simulink model "BuckyWagon_01"  (Simulink 7.5)
settings: Solver=FixedStepDiscrete  StartTime=0.0  StopTime=10.0  RelTol=1e-3
PreLoadFcn:
  | try, eval([bdroot '_setup']); catch, eval('model_setup', ''); end
InitFcn:
  | try, eval([bdroot '_setup']); catch, eval('model_setup', ''); end
undefined symbols (not defined in the file): ECU565, High, Low, miniviewSetup, motohawk_build_version, motohawk_get_faults, motohawk_setup_toolchains, motohawk_trunc_name, motohawk_vardec_config_group, motohawk_vardec_path, tc, True
libraries: MotoHawk_lib x381, simulink x26, miniview_lib x10, motohawk_control_primitives_lib x8, motohawk_engine_lib x6, motohawk_annotations_lib x2
(part 2 of 6)

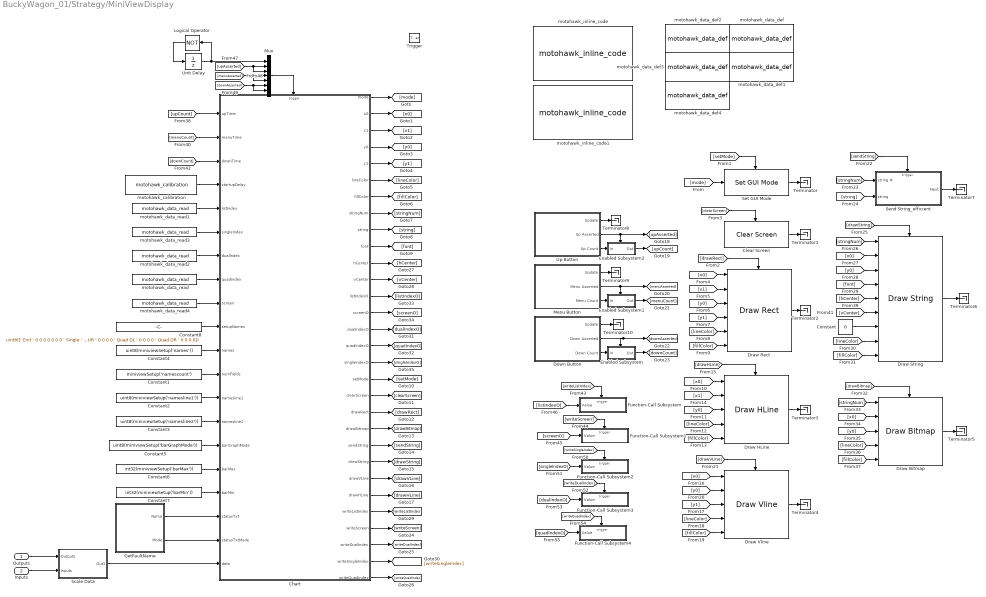
== system BuckyWagon_01/Strategy/MiniViewDisplay ==
  Outputs : Inport  OutDataType=sfix(16)  OutScaling=2^0
  Inputs : Inport  Port=2  OutDataType=sfix(16)  OutScaling=2^0
  Trigger : TriggerPort  TriggerType=function-call
  Chart : Stateflow chart  TreatAsAtomicUnit=on
      settings: RTWSystemCode=Reusable function
  Clear Screen : miniview_lib/Clear Screen  SystemSampleTime=-1  miniview_CAN_channel=1
  Constant : Constant  Value=0  OutDataType=sfix(16)  OutScaling=2^0  OutDataTypeStr=Inherit: Inherit via back propagation
  Constant1 : Constant  Value=miniviewSetup('namescount')  OutDataTypeMode=uint8  OutDataType=sfix(16)  OutScaling=2^0  OutDataTypeStr=uint8
  Constant2 : Constant  Value=uint8(miniviewSetup('namesline1'))  OutDataTypeMode=uint8  OutDataType=sfix(16)  OutScaling=2^0  OutDataTypeStr=uint8
  Constant3 : Constant  Value=uint8(miniviewSetup('namesline2'))  OutDataTypeMode=uint8  OutDataType=sfix(16)  OutScaling=2^0  OutDataTypeStr=uint8
  Constant4 : Constant  Value=uint8(miniviewSetup('names'))  OutDataTypeMode=uint8  OutDataType=sfix(16)  OutScaling=2^0  OutDataTypeStr=uint8
  Constant5 : Constant  Value=uint8(miniviewSetup('barGraphMode'))  OutDataTypeMode=uint8  OutDataType=sfix(16)  OutScaling=2^0  OutDataTypeStr=uint8
  Constant6 : Constant  Value=int32(miniviewSetup('barMax'))  OutDataTypeMode=int32  OutDataType=sfix(16)  OutScaling=2^0  OutDataTypeStr=int32
  Constant7 : Constant  Value=int32(miniviewSetup('barMin'))  OutDataTypeMode=int16  OutDataType=sfix(16)  OutScaling=2^0  OutDataTypeStr=int16
  Constant8 : Constant  Value=uint8([' Exit ' 0 0 0 0 0 0 0 ' Single ' 0 0 0 0 0 ' Dual Upper ' 0 ' Dual Lower ' 0 ' Quad UL ' 0 0 0 0 ' Quad UR ' 0 0 0 0 ' Quad DL ' 0 0 0 0 ' Quad DR ' 0 0 0 0])  OutDataTypeMode=uint8  OutDataType=sfix(16)  OutScaling=2^0  OutDataTypeStr=uint8
  Down Button : Subsystem  AncestorBlock=miniview_lib/Down Button  mask(MotoHawk MiniView Down Button){miniview_CAN_channel=1}
      mask prompts: miniview_CAN_channel "Physical CAN Channel"
      mask help: MotoHawk MiniView Down Button
      mask Display: disp(['MiniView "Down" Button\n\nChannel:  CAN_' num2str(miniview_CAN_channel)])
  Draw Bitmap : miniview_lib/Draw Bitmap  SystemSampleTime=-1  miniview_CAN_channel=1
  Draw HLine : miniview_lib/Draw HLine  SystemSampleTime=-1  miniview_CAN_channel=1
  Draw Rect : miniview_lib/Draw Rect  SystemSampleTime=-1  miniview_CAN_channel=1
  Draw String : miniview_lib/Draw String  SystemSampleTime=-1  miniview_CAN_channel=1
  Draw Vline : miniview_lib/Draw Vline  SystemSampleTime=-1  miniview_CAN_channel=1
  Enabled Subsystem : Subsystem  TreatAsAtomicUnit=on
  Enabled Subsystem1 : Subsystem  TreatAsAtomicUnit=on
  Enabled Subsystem2 : Subsystem  TreatAsAtomicUnit=on
  Function-Call Subsystem : Subsystem  TreatAsAtomicUnit=on
  Function-Call Subsystem1 : Subsystem  TreatAsAtomicUnit=on
  Function-Call Subsystem2 : Subsystem  TreatAsAtomicUnit=on
  Function-Call Subsystem3 : Subsystem  TreatAsAtomicUnit=on
  Function-Call Subsystem4 : Subsystem  TreatAsAtomicUnit=on
  GetFaultName : Subsystem
  Logical Operator : Logic  Operator=NOT  AllPortsSameDT=off  OutDataTypeMode=boolean  OutDataTypeStr=boolean
  Menu Button : Subsystem  AncestorBlock=miniview_lib/Menu Button  mask(MotoHawk MiniView Menu Button){miniview_CAN_channel=1}
      mask prompts: miniview_CAN_channel "Physical CAN Channel"
      mask help: MotoHawk MiniView Menu Button
      mask Display: disp(['MiniView "Menu" Button\n\nChannel:  CAN_' num2str(miniview_CAN_channel)])
  Mux : Mux  Inputs=7
  Scale Data : Subsystem
  Send String_efficient : Subsystem  AncestorBlock=miniview_lib/Send String  mask(MotoHawk MiniView Send String){miniview_CAN_channel=1}
      mask prompts: miniview_CAN_channel "Physical CAN Channel"
      mask help:
      | MotoHawk MiniView Send String
      |
      | Send string (#0 to #15) to gauge.
      mask Display: disp(['MiniView\nSend String\nChannel:  CAN_' num2str(miniview_CAN_channel)])
  Set GUI Mode : miniview_lib/Set GUI Mode  SystemSampleTime=-1  miniview_CAN_channel=1
  Terminator{,1..10} (11 alike) : Terminator
  Unit Delay : UnitDelay  SampleTime=-1
  Up Button : Subsystem  AncestorBlock=miniview_lib/Up Button  mask(MotoHawk MiniView Up Button){miniview_CAN_channel=1}
      mask prompts: miniview_CAN_channel "Physical CAN Channel"
      mask help: MotoHawk MiniView Up Button
      mask Display: disp(['MiniView "Up" Button\n\nChannel:  CAN_' num2str(miniview_CAN_channel)])
  motohawk_calibration : MotoHawk_lib/Calibration & Probing Blocks/motohawk_calibration  nam='startupDelay'  val=300  storage=Calibration  show_more=on  name_source=Use Parameter  data_type=uint16  read_level=1  write_level=1  ovr_cals=on  view_as=Number  enum_struct={'Disabled', 'Enabled'}  vector_style=Wide Row  use_help_units=on  help='Time to wait before drawing on the miniview.'  units='s'  use_header_enum=off  row_header_enum={}  col_header_enum={}  use_min_max=on  min_val=0  max_val=10  use_precision=on  precision='1.3'  gain=0.005  offset=0  exp=1  use_mototune_group=off  mototune_group=motohawk_vardec_path(gcb)
  motohawk_data_def : MotoHawk_lib/Data Storage Blocks/motohawk_data_def  nam='quadIndex'  container_nam=''  data=[0 5 16 19]  typ=uint8  struct_nam='MyStruct'  storage=NonVolatile  outputRef=off  use_vardec=on  window=Display  read_level=1  write_level=1  ovr_cals=on  view_as=Number  enum_struct={'Disabled', 'Enabled'}  vector_style=Tall Column  use_help_units=on  help=''  units=''  use_header_enum=off  row_header_enum=''  col_header_enum=''  use_min_max=off  min_val=-inf  max_val=inf  use_precision=off  precision=''  gain=1  offset=0  exp=1  use_mototune_group=off  mototune_group=motohawk_vardec_path(gcb)  eval_name=quadIndex  data_stores=motohawk_sfun_data_def_data_stores  struct_instances=motohawk_sfun_data_def_struct_instances  vardecs=motohawk_sfun_data_def_vardecs
  motohawk_data_def1 : MotoHawk_lib/Data Storage Blocks/motohawk_data_def  nam='listIndex'  container_nam=''  data=0  typ=uint8  struct_nam='MyStruct'  storage=NonVolatile  outputRef=off  use_vardec=on  window=Display  read_level=1  write_level=1  ovr_cals=on  view_as=Number  enum_struct={'Disabled', 'Enabled'}  vector_style=Tall Column  use_help_units=on  help=''  units=''  use_header_enum=off  row_header_enum=''  col_header_enum=''  use_min_max=off  min_val=-inf  max_val=inf  use_precision=off  precision=''  gain=1  offset=0  exp=1  use_mototune_group=off  mototune_group=motohawk_vardec_path(gcb)  eval_name=listIndex  data_stores=motohawk_sfun_data_def_data_stores  struct_instances=motohawk_sfun_data_def_struct_instances  vardecs=motohawk_sfun_data_def_vardecs
  motohawk_data_def2 : MotoHawk_lib/Data Storage Blocks/motohawk_data_def  nam='dualIndex'  container_nam=''  data=[10 27]  typ=uint8  struct_nam='MyStruct'  storage=NonVolatile  outputRef=off  use_vardec=on  window=Display  read_level=1  write_level=1  ovr_cals=on  view_as=Number  enum_struct={'Disabled', 'Enabled'}  vector_style=Tall Column  use_help_units=on  help=''  units=''  use_header_enum=off  row_header_enum=''  col_header_enum=''  use_min_max=off  min_val=-inf  max_val=inf  use_precision=off  precision=''  gain=1  offset=0  exp=1  use_mototune_group=off  mototune_group=motohawk_vardec_path(gcb)  eval_name=dualIndex  data_stores=motohawk_sfun_data_def_data_stores  struct_instances=motohawk_sfun_data_def_struct_instances  vardecs=motohawk_sfun_data_def_vardecs
  motohawk_data_def3 : MotoHawk_lib/Data Storage Blocks/motohawk_data_def  nam='singleIndex'  container_nam=''  data=15  typ=uint8  struct_nam='MyStruct'  storage=NonVolatile  outputRef=off  use_vardec=on  window=Display  read_level=1  write_level=1  ovr_cals=on  view_as=Number  enum_struct={'Disabled', 'Enabled'}  vector_style=Tall Column  use_help_units=on  help=''  units=''  use_header_enum=off  row_header_enum=''  col_header_enum=''  use_min_max=off  min_val=-inf  max_val=inf  use_precision=off  precision=''  gain=1  offset=0  exp=1  use_mototune_group=off  mototune_group=motohawk_vardec_path(gcb)  eval_name=singleIndex  data_stores=motohawk_sfun_data_def_data_stores  struct_instances=motohawk_sfun_data_def_struct_instances  vardecs=motohawk_sfun_data_def_vardecs
  motohawk_data_def4 : MotoHawk_lib/Data Storage Blocks/motohawk_data_def  nam='screen'  container_nam=''  data=0  typ=uint8  struct_nam='MyStruct'  storage=NonVolatile  outputRef=off  use_vardec=on  window=Display  read_level=1  write_level=1  ovr_cals=on  view_as=Number  enum_struct={'Disabled', 'Enabled'}  vector_style=Tall Column  use_help_units=on  help=''  units=''  use_header_enum=off  row_header_enum=''  col_header_enum=''  use_min_max=off  min_val=-inf  max_val=inf  use_precision=off  precision=''  gain=1  offset=0  exp=1  use_mototune_group=off  mototune_group=motohawk_vardec_path(gcb)  eval_name=screen  data_stores=motohawk_sfun_data_def_data_stores  struct_instances=motohawk_sfun_data_def_struct_instances  vardecs=motohawk_sfun_data_def_vardecs
  motohawk_data_read : MotoHawk_lib/Data Storage Blocks/motohawk_data_read  source=Lookup By Name  structure=Vector  operation=Read entire data structure at once  sz_vec=4  sz_row=2  sz_col=3  typ=uint8  nam='quadIndex'  checkNull=on  struct_inst_name='Struct1'  struct_nam='MyStruct'
  motohawk_data_read1 : MotoHawk_lib/Data Storage Blocks/motohawk_data_read  source=Lookup By Name  structure=Scalar  operation=Read scalar from location by index  sz_vec=4  sz_row=2  sz_col=3  typ=uint8  nam='listIndex'  checkNull=on  struct_inst_name='Struct1'  struct_nam='MyStruct'
  motohawk_data_read2 : MotoHawk_lib/Data Storage Blocks/motohawk_data_read  source=Lookup By Name  structure=Vector  operation=Read entire data structure at once  sz_vec=2  sz_row=2  sz_col=3  typ=uint8  nam='dualIndex'  checkNull=on  struct_inst_name='Struct1'  struct_nam='MyStruct'
  motohawk_data_read3 : MotoHawk_lib/Data Storage Blocks/motohawk_data_read  source=Lookup By Name  structure=Scalar  operation=Read scalar from location by index  sz_vec=4  sz_row=2  sz_col=3  typ=uint8  nam='singleIndex'  checkNull=on  struct_inst_name='Struct1'  struct_nam='MyStruct'
  motohawk_data_read4 : MotoHawk_lib/Data Storage Blocks/motohawk_data_read  source=Lookup By Name  structure=Scalar  operation=Read entire data structure at once  sz_vec=4  sz_row=2  sz_col=3  typ=uint8  nam='screen'  checkNull=on  struct_inst_name='Struct1'  struct_nam='MyStruct'
  motohawk_inline_code : MotoHawk_lib/Extra Development Blocks/motohawk_inline_code  include_code='#include <stdio.h>'  start_code=''  output_code=''
  motohawk_inline_code1 : MotoHawk_lib/Extra Development Blocks/motohawk_inline_code  include_code='#define charPtr(p) ((char*)p)'  start_code=''  output_code=''
  wires:
  Outputs/1 -> Scale Data/1(Outputs)
  Inputs/1 -> Scale Data/2(Inputs)
  Chart/1(mode) -> [mode]
  Chart/2(x0) -> [x0]
  Chart/3(x1) -> [x1]
  Chart/4(y0) -> [y0]
  Chart/5(y1) -> [y1]
  Chart/6(lineColor) -> [lineColor]
  Chart/7(fillColor) -> [fillColor]
  Chart/8(stringNum) -> [stringNum]
  Chart/9(string) -> [string]
  Chart/10(font) -> [font]
  Chart/19(clearScreen) -> [clearScreen]
  Chart/20(drawRect) -> [drawRect]
  Chart/21(drawBitmap) -> [drawBitmap]
  Chart/22(sendString) -> [sendString]
  Chart/23(drawString) -> [drawString]
  Chart/24(drawVLine) -> [drawVLine]
  Chart/25(drawHLine) -> [drawHLine]
  [setMode] -> Set GUI Mode/Trigger
  [mode] -> Set GUI Mode/1
  Set GUI Mode/1 -> Terminator/1
  [clearScreen] -> Clear Screen/Trigger
  Clear Screen/1 -> Terminator1/1
  [drawRect] -> Draw Rect/Trigger
  [x0] -> Draw Rect/1
  [x1] -> Draw Rect/2
  [y0] -> Draw Rect/3
  [y1] -> Draw Rect/4
  [lineColor] -> Draw Rect/5
  [fillColor] -> Draw Rect/6
  [x0] -> Draw HLine/1
  [x1] -> Draw HLine/2
  [y0] -> Draw HLine/3
  [lineColor] -> Draw HLine/4
  [fillColor] -> Draw HLine/5
  [drawHLine] -> Draw HLine/Trigger
  [x0] -> Draw Vline/1
  [y0] -> Draw Vline/2
  [y1] -> Draw Vline/3
  [lineColor] -> Draw Vline/4
  [fillColor] -> Draw Vline/5
  [drawVLine] -> Draw Vline/Trigger
  Draw Rect/1 -> Terminator2/1
  Draw Vline/1 -> Terminator4/1
  Draw HLine/1 -> Terminator3/1
  [sendString] -> Send String_efficient/Trigger
  [stringNum] -> Send String_efficient/1(string #)
  [string] -> Send String_efficient/2(string)
  [drawString] -> Draw String/Trigger
  [stringNum] -> Draw String/1
  [x0] -> Draw String/2
  [y0] -> Draw String/3
  [font] -> Draw String/4
  [lineColor] -> Draw String/8
  [fillColor] -> Draw String/9
  [drawBitmap] -> Draw Bitmap/Trigger
  [stringNum] -> Draw Bitmap/1
  [x0] -> Draw Bitmap/2
  [y0] -> Draw Bitmap/3
  [lineColor] -> Draw Bitmap/4
  [fillColor] -> Draw Bitmap/5
  Draw Bitmap/1 -> Terminator5/1
  Draw String/1 -> Terminator6/1
  Send String_efficient/1(Next) -> Terminator7/1
  [upCount] -> Chart/1(upTime)
  [menuCount] -> Chart/2(menuTime)
  [downCount] -> Chart/3(downTime)
  Up Button/2(Up Asserted) -> [upAsserted], Enabled Subsystem2/Enable
  Down Button/2(Down Asserted) -> [downAsserted], Enabled Subsystem/Enable
  Menu Button/2(Menu Asserted) -> [menuAsserted], Enabled Subsystem1/Enable
  [upAsserted] -> Mux/2, Mux/3
  [menuAsserted] -> Mux/4, Mux/5
  [downAsserted] -> Mux/6, Mux/7
  Mux/1 -> Chart/Trigger
  Constant/1 -> Draw String/7
  [hCenter] -> Draw String/5
  [vCenter] -> Draw String/6
  Chart/11(hCenter) -> [hCenter]
  Chart/12(vCenter) -> [vCenter]
  Unit Delay/1 -> Mux/1, Logical Operator/1
  Constant4/1 -> Chart/11(names)
  Logical Operator/1 -> Unit Delay/1
  Scale Data/1(Out1) -> Chart/20(data)
  Constant2/1 -> Chart/13(namesline1)
  Constant3/1 -> Chart/14(namesline2)
  motohawk_data_read1/1 -> Chart/5(listIndex)
  motohawk_data_read/1 -> Chart/8(quadIndex)
  Chart/26(writeListIndex) -> [writeListIndex]
  [writeListIndex] -> Function-Call Subsystem/Trigger
  motohawk_data_read2/1 -> Chart/7(dualIndex)
  motohawk_data_read3/1 -> Chart/6(singleIndex)
  Constant5/1 -> Chart/15(barGraphMode)
  Constant6/1 -> Chart/16(barMax)
  Constant7/1 -> Chart/17(barMin)
  Up Button/1(Update) -> Terminator8/1
  Menu Button/1(Update) -> Terminator9/1
  Down Button/1(Update) -> Terminator10/1
  Constant8/1 -> Chart/10(setupNames)
  Chart/27(writeScreen) -> [writeScreen]
  [writeScreen] -> Function-Call Subsystem1/Trigger
  motohawk_data_read4/1 -> Chart/9(screen)
  Down Button/3(Down Count) -> Enabled Subsystem/1(In)
  Enabled Subsystem/1(Out) -> [downCount]
  Menu Button/3(Menu Count) -> Enabled Subsystem1/1(In)
  Enabled Subsystem1/1(Out) -> [menuCount]
  Up Button/3(Up Count) -> Enabled Subsystem2/1(In)
  Enabled Subsystem2/1(Out) -> [upCount]
  Chart/28(writeDualIndex) -> [writeDualIndex]
  Chart/29(writeSingleIndex) -> [writeSingleIndex]
  Chart/30(writeQuadIndex) -> [writeQuadIndex]
  Chart/13(listIndexO) -> [listIndexO]
  Chart/14(screenO) -> [screenO]
  Chart/15(dualIndexO) -> [dualIndexO]
  Chart/16(quadIndexO) -> [quadIndexO]
  Chart/17(singleIndexO) -> [singleIndexO]
  [screenO] -> Function-Call Subsystem1/1(Value)
  [listIndexO] -> Function-Call Subsystem/1(Value)
  [writeSingleIndex] -> Function-Call Subsystem2/Trigger
  [singleIndexO] -> Function-Call Subsystem2/1(Value)
  [writeDualIndex] -> Function-Call Subsystem3/Trigger
  [dualIndexO] -> Function-Call Subsystem3/1(Value)
  [writeQuadIndex] -> Function-Call Subsystem4/Trigger
  [quadIndexO] -> Function-Call Subsystem4/1(Value)
  Constant1/1 -> Chart/12(numFields)
  Chart/18(setMode) -> [setMode]
  GetFaultName/1(Name) -> Chart/18(statusTxt)
  GetFaultName/2(Mode) -> Chart/19(statusTxtMode)
  motohawk_calibration/1 -> Chart/4(startupDelay)

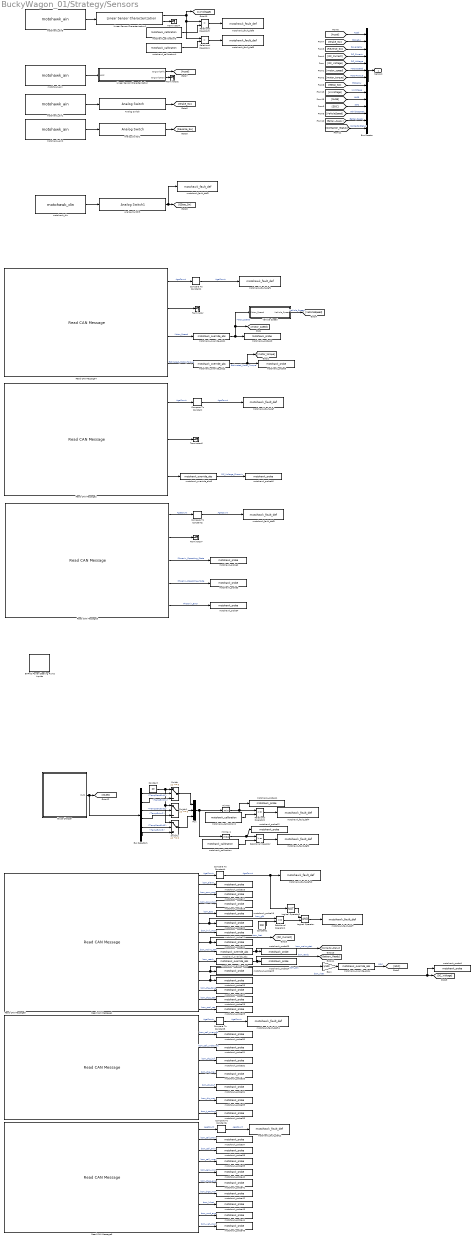
== system BuckyWagon_01/Strategy/Sensors ==
  Analog Switch : motohawk_engine_lib/Analog Switch  SystemSampleTime=-1  nam='Brake_Switch'  prefix='Brake_'  switchpoint=500  polarity=High-True  parent_group='Sensors | Brake'
  Analog Switch1 : motohawk_engine_lib/Analog Switch  SystemSampleTime=-1  nam='Reverse_Switch'  prefix='Reverse_'  switchpoint=500  polarity=Low-True  parent_group='Sensors | Reverse'
  Analog Switch3 : motohawk_engine_lib/Analog Switch1  SystemSampleTime=-1  nam='EStop_Switch'  prefix='EStop_'  polarity=Low-True  parent_group='Sensors | EStop'
  Brusa Charger : Subsystem  AncestorBlock=motohawk_annotations_lib/Display Image File  mask(Display Image File){image_file='NLG5.jpg'}
      mask prompts: image_file "Image File"
      mask help:
      | Enter an image file on the current MATLAB path to display on this block.
      |
      | Double-clicking this block opens the contents of the subsystem.  Right-click and select 'Mask parameters...' to select a new image file.
      |
      | To use just the mask of this block in a model, but supply your own contents, break the link to the library.
      mask init:
      | try,
      | 	img = imread(image_file);
      | 	motohawk_block_image(gcb, image_file);
      | catch,
      | 	img = imread('image_not_found.jpg');
      | end
      settings: OpenFcn=open_system(gcb,'force');  MoveFcn=motohawk_block_image(gcb, motohawk_get_param_ws(gcb, 'image_file'));
      mask Display: image(img);
  Bus Creator : BusCreator  Inputs=14
  Bus Selector1 : BusSelector  OutputSignals=Errors/Warnings.TempSensExt1,Temp.TempExtrn1,Errors/Warnings.TempSensExt2,Temp.TempExtrn2,Errors/Warnings.TempSensExt3,Temp.TempExtrn3
  Compare To Constant{,1..2,4..6} (6 alike) : simulink/Logic and Bit Operations/Compare To Constant  SystemSampleTime=-1  relop=>  const=50/5*2  LogicOutDataTypeMode=boolean  ZeroCross=off
  Constant : Constant  Value=20  OutDataType=sfix(16)  OutScaling=2^0
  Constant1 : Constant  Value=200  OutDataType=fixdt(1, 16)  OutScaling=2^0
  EHPAS Power Steering Pump Inputts : Subsystem  TreatAsAtomicUnit=on
  Gain : Gain  Gain=1/100  ParameterDataType=fixdt(1, 16)  ParameterScaling=2^0  OutDataType=fixdt(1, 16)  OutScaling=2^0
  Linear Sensor Characterization : Subsystem  AncestorBlock=motohawk_engine_lib/Linear Sensor Characterization  mask(Linear Sensor Characterization){nam='Accel_Pedal', prefix='Accel_', units='%', inputunits='ADC', parent_group='Sensors | Accel', samp_time=0.005}
      mask prompts: nam "Name"; units "Output Units"; inputunits "Input Units"; parent_group "MotoTune Group"; samp_time "Sample Time"
      mask help:
      | Converts from A/D Counts to Engineering Units, using a Gain and Offset.
      | Saturates the converted value around Min and Max values, and triggers a Fault when out of range.
      mask init:
      | lbl = ['Linear Sensor: ' nam ' [' units ']'];
      | group = [parent_group ' | ' nam];
      settings: RTWSystemCode=Function  RTWFcnNameOpts=Use subsystem name  RTWFileNameOpts=Use function name
      mask Display:
      | patch([0 0 1 1], [0 0.075 0.075 0], [230/255 0/255 0/255])
      | patch([0 0 1 1], [0.025 0.05 0.05 0.025], [150/255 0/255 0/255])
      | patch([0 0 1 1], [0 0.025 0.025 0], [0/255 0/255 0/255])
      | 
      | disp(lbl);
  Linear Sensor Characterization1 : motohawk_engine_lib/Linear Sensor Characterization  SystemSampleTime=-1  nam='LVVolt'  prefix='LVVolt_'  units='V'  inputunits='ADC'  parent_group='Sensors | LVVolt'  samp_time=0.005
      link override First Order Low Pass/motohawk_calibration: val=0.005
      link override motohawk_fault_def2: id=0
      link override motohawk_fault_def3: id=0
  Logical Operator : Logic  AllPortsSameDT=off  OutDataTypeMode=boolean  LogicDataType=fixdt(0, 8)  OutDataTypeStr=boolean
  Logical Operator1 : Logic  Operator=NOT  Inputs=1  AllPortsSameDT=off  OutDataTypeMode=boolean  LogicDataType=fixdt(0, 8)  OutDataTypeStr=boolean
  MinMax : MinMax  OutDataType=sfix(16)  OutScaling=2^0
  MinMax1 : MinMax  Function=max  OutDataType=sfix(16)  OutScaling=2^0
  Mux : Mux  Inputs=3
  Read CAN Message1 : MotoHawk_lib/CAN Blocks/Read CAN Message  nam='CAN_2'  bus=-2  msg=BMS_A123_410  queue=1  slot=''  valid=off  stale=on  labelwires=on
  Read CAN Message2 : MotoHawk_lib/CAN Blocks/Read CAN Message  nam='CAN_1'  bus=-2  msg=J1939_F9_Status3  queue=1  slot=''  valid=off  stale=on  labelwires=off
  Read CAN Message3 : MotoHawk_lib/CAN Blocks/Read CAN Message  nam='CAN_1'  bus=-2  msg=J1939_F9_Status2  queue=1  slot=''  valid=off  stale=on  labelwires=off
  Read CAN Message4 : MotoHawk_lib/CAN Blocks/Read CAN Message  nam='CAN_1'  bus=-2  msg=J1939_F9_Status1  queue=1  slot=''  valid=off  stale=on  labelwires=off
  Read CAN Message5 : MotoHawk_lib/CAN Blocks/Read CAN Message  nam='CAN_2'  bus=-2  msg=BMS_A123_420  queue=1  slot=''  valid=off  stale=on  labelwires=on
  Read CAN Message6 : MotoHawk_lib/CAN Blocks/Read CAN Message  nam='CAN_2'  bus=-2  msg=BMS_A123_430  queue=1  slot=''  valid=off  stale=on  labelwires=on
  Relational Operator : RelationalOperator  LogicOutDataTypeMode=boolean  OutDataTypeStr=boolean
  Relational Operator1 : RelationalOperator  Operator=<=  LogicOutDataTypeMode=boolean  LogicDataType=fixdt(0, 8)  OutDataTypeStr=boolean
  Relational Operator2 : RelationalOperator  Operator=<=  LogicOutDataTypeMode=boolean  OutDataTypeStr=boolean
  Relational Operator3 : RelationalOperator  Operator=<  LogicOutDataTypeMode=boolean  OutDataTypeStr=boolean
  Relational Operator4 : RelationalOperator  Operator=>  LogicOutDataTypeMode=boolean  OutDataTypeStr=boolean
  Switch : Switch  Criteria=u2 ~= 0  OutDataType=sfix(16)  OutScaling=2^0
  Switch1 : Switch  Criteria=u2 ~= 0  OutDataType=sfix(16)  OutScaling=2^0
  Switch2 : Switch  Criteria=u2 ~= 0  OutDataType=sfix(16)  OutScaling=2^0
  Terminator{,2,4,6..7} (5 alike) : Terminator
  Vehicle Speed : Subsystem
  motohawk_ain : MotoHawk_lib/Analog I//O Blocks/motohawk_ain  res_name=[]  text_resource=AN4M  code_resource=NONE  val_resource=-1  target=ECU565-128  resource_enum_str=(None)=-1,ECUP=53,DRVP=54,XDRP=55,AN1M=56,AN2M=57,AN3M=58,AN4M=59,AN5M=60,AN6M=61,AN7M=62,AN8M=63,AN9M=64,AN10M=65,AN11M=66,AN12M=67,AN13M=68,AN14M=69,AN15M=70,AN16M=71,AN17M=72,AN18M=73,AN19M=74,AN20M=75,AN21M=76,AN22M=77,AN23M=78,AN24M=79,AN25M=80,AN26M=81,AN27M=82,AN28M=83,AN29M=84,AN30M=85,AN31M=86,AN32M=87,AN33M=88,AN34M=89,O2A=90,O2B=91,XDRP_B=92,REF_14V=143  altref=5V Reference  typ=uint16  num_adc_bits=10  use_stat=off  use_vardec=on  nam='Accel_Pedal_Pin'  read_level=1  write_level=1  group='System | I/O Pins | Inputs Config'
  motohawk_ain1 : MotoHawk_lib/Analog I//O Blocks/motohawk_ain  res_name=[]  text_resource=AN2M  code_resource=NONE  val_resource=-1  target=ECU565-128  resource_enum_str=(None)=-1,ECUP=53,DRVP=54,XDRP=55,AN1M=56,AN2M=57,AN3M=58,AN4M=59,AN5M=60,AN6M=61,AN7M=62,AN8M=63,AN9M=64,AN10M=65,AN11M=66,AN12M=67,AN13M=68,AN14M=69,AN15M=70,AN16M=71,AN17M=72,AN18M=73,AN19M=74,AN20M=75,AN21M=76,AN22M=77,AN23M=78,AN24M=79,AN25M=80,AN26M=81,AN27M=82,AN28M=83,AN29M=84,AN30M=85,AN31M=86,AN32M=87,AN33M=88,AN34M=89,O2A=90,O2B=91,XDRP_B=92,REF_14V=143  altref=5V Reference  typ=uint16  num_adc_bits=10  use_stat=off  use_vardec=on  nam='Brake_Switch_Pin'  read_level=1  write_level=1  group='System | I/O Pins | Inputs Config'
  motohawk_ain2 : MotoHawk_lib/Analog I//O Blocks/motohawk_ain  res_name=[]  text_resource=AN1M  code_resource=NONE  val_resource=-1  target=ECU565-128  resource_enum_str=(None)=-1,ECUP=53,DRVP=54,XDRP=55,AN1M=56,AN2M=57,AN3M=58,AN4M=59,AN5M=60,AN6M=61,AN7M=62,AN8M=63,AN9M=64,AN10M=65,AN11M=66,AN12M=67,AN13M=68,AN14M=69,AN15M=70,AN16M=71,AN17M=72,AN18M=73,AN19M=74,AN20M=75,AN21M=76,AN22M=77,AN23M=78,AN24M=79,AN25M=80,AN26M=81,AN27M=82,AN28M=83,AN29M=84,AN30M=85,AN31M=86,AN32M=87,AN33M=88,AN34M=89,O2A=90,O2B=91,XDRP_B=92,REF_14V=143  altref=5V Reference  typ=uint16  num_adc_bits=10  use_stat=off  use_vardec=on  nam='Reverse_Switch_Pin'  read_level=1  write_level=1  group='System | I/O Pins | Inputs Config'
  motohawk_ain5 : MotoHawk_lib/Analog I//O Blocks/motohawk_ain  res_name=[]  text_resource=DRVP  code_resource=NONE  val_resource=-1  target=ECU565-128  resource_enum_str=(None)=-1,ECUP=53,DRVP=54,XDRP=55,AN1M=56,AN2M=57,AN3M=58,AN4M=59,AN5M=60,AN6M=61,AN7M=62,AN8M=63,AN9M=64,AN10M=65,AN11M=66,AN12M=67,AN13M=68,AN14M=69,AN15M=70,AN16M=71,AN17M=72,AN18M=73,AN19M=74,AN20M=75,AN21M=76,AN22M=77,AN23M=78,AN24M=79,AN25M=80,AN26M=81,AN27M=82,AN28M=83,AN29M=84,AN30M=85,AN31M=86,AN32M=87,AN33M=88,AN34M=89,O2A=90,O2B=91,XDRP_B=92,REF_14V=143  altref=5V Reference  typ=uint16  num_adc_bits=10  use_stat=off  use_vardec=on  nam='LV_Voltage_Pin'  read_level=1  write_level=1  group='System | I/O Pins | Inputs Config'
  motohawk_calibration : MotoHawk_lib/Calibration & Probing Blocks/motohawk_calibration  nam='BattOverTemp_Pt'  val=70  storage=Calibration  show_more=on  name_source=Use Parameter  data_type=Inherit from 'Default Value'  read_level=1  write_level=1  ovr_cals=on  view_as=Number  enum_struct={'Disabled', 'Enabled'}  vector_style=Wide Row  use_help_units=on  help='Temperature at which an overtemp fault occurs'  units='C'  use_header_enum=off  row_header_enum={}  col_header_enum={}  use_min_max=off  min_val=-inf  max_val=inf  use_precision=off  precision=''  gain=1  offset=0  exp=1  use_mototune_group=on  mototune_group='Sensors | Brusa'
  motohawk_calibration2 : MotoHawk_lib/Calibration & Probing Blocks/motohawk_calibration  nam='BattUnderTemp_Pt'  val=-40  storage=Calibration  show_more=on  name_source=Use Parameter  data_type=Inherit from 'Default Value'  read_level=1  write_level=1  ovr_cals=on  view_as=Number  enum_struct={'Disabled', 'Enabled'}  vector_style=Wide Row  use_help_units=on  help='Temperature at which an overtemp fault occurs'  units='C'  use_header_enum=off  row_header_enum={}  col_header_enum={}  use_min_max=off  min_val=-inf  max_val=inf  use_precision=off  precision=''  gain=1  offset=0  exp=1  use_mototune_group=on  mototune_group='Sensors | Brusa'
  motohawk_calibration3 : MotoHawk_lib/Calibration & Probing Blocks/motohawk_calibration  nam='Low12VThres'  val=12.8  storage=Calibration  show_more=on  name_source=Use Parameter  data_type=Inherit from 'Default Value'  read_level=1  write_level=1  ovr_cals=on  view_as=Number  enum_struct={'Disabled', 'Enabled'}  vector_style=Wide Row  use_help_units=on  help='Voltage below with low 12V fault occurs.'  units='V'  use_header_enum=off  row_header_enum={}  col_header_enum={}  use_min_max=off  min_val=-inf  max_val=inf  use_precision=on  precision=''  gain=1  offset=0  exp=1  use_mototune_group=on  mototune_group='Sensors | LVVolt'
  motohawk_calibration4 : MotoHawk_lib/Calibration & Probing Blocks/motohawk_calibration  nam='High12VThres'  val=14.5  storage=Calibration  show_more=on  name_source=Use Parameter  data_type=Inherit from 'Default Value'  read_level=1  write_level=1  ovr_cals=on  view_as=Number  enum_struct={'Disabled', 'Enabled'}  vector_style=Wide Row  use_help_units=on  help='Voltage below with low 12V fault occurs.'  units='V'  use_header_enum=off  row_header_enum={}  col_header_enum={}  use_min_max=off  min_val=-inf  max_val=inf  use_precision=on  precision=''  gain=1  offset=0  exp=1  use_mototune_group=on  mototune_group='Sensors | LVVolt'
  motohawk_din : MotoHawk_lib/Digital I//O Blocks/motohawk_din  resource_name=[]  text_resource=(None)  code_resource=RES_AN1M  val_resource=-1  target=ECU565-128  resource_enum_str=(None)=-1,AN1M=56,AN2M=57,AN3M=58,AN4M=59,AN5M=60,AN6M=61,AN7M=62,AN8M=63,AN9M=64,AN10M=65,AN11M=66,AN12M=67,AN13M=68,AN14M=69,AN15M=70,AN16M=71,AN17M=72,AN18M=73,AN19M=74,AN20M=75,AN21M=76,AN22M=77,AN23M=78,AN24M=79,AN25M=80,AN26M=81,AN27M=82,AN28M=83,AN29M=84,AN30M=85,AN31M=86,AN32M=87,AN33M=88,AN34M=89,O2A=90,O2B=91,DG1M=93,DG2M=94,DG3M=95,DG4M=96,DG5M=102,DG6M=103,DG7M=104,SPD1=105,SPD2=106,DG8M=111  pullup=None  use_stat=off  use_vardec=on  nam='EStop_Switch_Pin'  read_level=1  write_level=1  group='System | I/O Pins | Inputs Config'
  motohawk_fault_def : MotoHawk_lib/Fault Management Blocks/motohawk_fault_def  nam='Phoenix_NoCAN_Status_3'  mode=Enabled  id=0  x=10  y=20  input_suspected=on  indeterminate=off  increment_xy=on  downsample_count=1  ovr_cals=on  ovr_actions=on  show_actions=off  action1_name=''  action1_cond=(None)  action2_name=''  action2_cond=(None)  action3_name=''  action3_cond=(None)  action4_name=''  action4_cond=(None)
  motohawk_fault_def1 : MotoHawk_lib/Fault Management Blocks/motohawk_fault_def  nam='Phoenix_NoCAN_Status_1'  mode=Enabled  id=0  x=10  y=20  input_suspected=on  indeterminate=off  increment_xy=on  downsample_count=1  ovr_cals=on  ovr_actions=on  show_actions=off  action1_name=''  action1_cond=(None)  action2_name=''  action2_cond=(None)  action3_name=''  action3_cond=(None)  action4_name=''  action4_cond=(None)
  motohawk_fault_def10 : MotoHawk_lib/Fault Management Blocks/motohawk_fault_def  nam='BCM_NoCAN410_Status'  mode=Enabled  id=0  x=10  y=20  input_suspected=on  indeterminate=off  increment_xy=on  downsample_count=1  ovr_cals=on  ovr_actions=on  show_actions=off  action1_name=''  action1_cond=(None)  action2_name=''  action2_cond=(None)  action3_name=''  action3_cond=(None)  action4_name=''  action4_cond=(None)
  motohawk_fault_def11 : MotoHawk_lib/Fault Management Blocks/motohawk_fault_def  nam='BCM_NoCAN420_Status'  mode=Enabled  id=0  x=10  y=20  input_suspected=on  indeterminate=off  increment_xy=on  downsample_count=1  ovr_cals=on  ovr_actions=on  show_actions=off  action1_name=''  action1_cond=(None)  action2_name=''  action2_cond=(None)  action3_name=''  action3_cond=(None)  action4_name=''  action4_cond=(None)
  motohawk_fault_def12 : MotoHawk_lib/Fault Management Blocks/motohawk_fault_def  nam='BCM_NoCAN430_Status'  mode=Enabled  id=0  x=10  y=20  input_suspected=on  indeterminate=off  increment_xy=on  downsample_count=1  ovr_cals=on  ovr_actions=on  show_actions=off  action1_name=''  action1_cond=(None)  action2_name=''  action2_cond=(None)  action3_name=''  action3_cond=(None)  action4_name=''  action4_cond=(None)
  motohawk_fault_def2 : MotoHawk_lib/Fault Management Blocks/motohawk_fault_def  nam='BattOverTemp'  mode=Disabled  id=0  x=25  y=50  input_suspected=on  indeterminate=off  increment_xy=on  downsample_count=1  ovr_cals=on  ovr_actions=on  show_actions=off  action1_name=''  action1_cond=(None)  action2_name=''  action2_cond=(None)  action3_name=''  action3_cond=(None)  action4_name=''  action4_cond=(None)
  motohawk_fault_def3 : MotoHawk_lib/Fault Management Blocks/motohawk_fault_def  nam='ESTOPped'  mode=Enabled  id=0  x=10  y=20  input_suspected=on  indeterminate=off  increment_xy=on  downsample_count=1  ovr_cals=on  ovr_actions=on  show_actions=off  action1_name=''  action1_cond=(None)  action2_name=''  action2_cond=(None)  action3_name=''  action3_cond=(None)  action4_name=''  action4_cond=(None)
  motohawk_fault_def4 : MotoHawk_lib/Fault Management Blocks/motohawk_fault_def  nam='BattUnderTemp'  mode=Disabled  id=0  x=25  y=50  input_suspected=on  indeterminate=off  increment_xy=on  downsample_count=1  ovr_cals=on  ovr_actions=on  show_actions=off  action1_name=''  action1_cond=(None)  action2_name=''  action2_cond=(None)  action3_name=''  action3_cond=(None)  action4_name=''  action4_cond=(None)
  motohawk_fault_def5 : MotoHawk_lib/Fault Management Blocks/motohawk_fault_def  nam='LVVoltLow'  mode=Enabled  id=0  x=100  y=200  input_suspected=on  indeterminate=off  increment_xy=on  downsample_count=1  ovr_cals=on  ovr_actions=on  show_actions=off  action1_name=''  action1_cond=(None)  action2_name=''  action2_cond=(None)  action3_name=''  action3_cond=(None)  action4_name=''  action4_cond=(None)
  motohawk_fault_def6 : MotoHawk_lib/Fault Management Blocks/motohawk_fault_def  nam='LVVoltHigh'  mode=Enabled  id=0  x=25  y=50  input_suspected=on  indeterminate=off  increment_xy=on  downsample_count=1  ovr_cals=on  ovr_actions=on  show_actions=off  action1_name=''  action1_cond=(None)  action2_name=''  action2_cond=(None)  action3_name=''  action3_cond=(None)  action4_name=''  action4_cond=(None)
  motohawk_fault_def7 : MotoHawk_lib/Fault Management Blocks/motohawk_fault_def  nam='GroundFlt'  mode=Enabled - Persistent  id=0  x=25  y=50  input_suspected=on  indeterminate=off  increment_xy=on  downsample_count=1  ovr_cals=on  ovr_actions=on  show_actions=off  action1_name='EmergencyShutdown'  action1_cond=Active  action2_name=''  action2_cond=(None)  action3_name=''  action3_cond=(None)  action4_name=''  action4_cond=(None)
  motohawk_fault_def9 : MotoHawk_lib/Fault Management Blocks/motohawk_fault_def  nam='Phoenix_NoCAN_Status_2'  mode=Enabled  id=0  x=10  y=20  input_suspected=on  indeterminate=off  increment_xy=on  downsample_count=1  ovr_cals=on  ovr_actions=on  show_actions=off  action1_name=''  action1_cond=(None)  action2_name=''  action2_cond=(None)  action3_name=''  action3_cond=(None)  action4_name=''  action4_cond=(None)
  motohawk_override_abs : MotoHawk_lib/Calibration & Probing Blocks/motohawk_override_abs  SystemSampleTime=-1  parent_name='bcm_mainc_stat'  parent_val=0  show_more=on  name_source=Use Parameter  parent_read_level=1  parent_override_level=1  view_as=Number  enum_struct={'Disabled', 'Enabled'}  use_help_units=off  parent_help=''  parent_units=''  use_min_max=off  parent_min=-inf  parent_max=inf  use_precision=off  parent_precision=''  parent_gain=1  parent_offset=0  parent_exp=1  use_mototune_group=on  parent_group='Sensors | BCM'
  motohawk_override_abs1 : MotoHawk_lib/Calibration & Probing Blocks/motohawk_override_abs  SystemSampleTime=-1  parent_name='Override_Absolute'  parent_val=0  show_more=on  name_source=Use Input Wire Name  parent_read_level=1  parent_override_level=1  view_as=Number  enum_struct={'Disabled', 'Enabled'}  use_help_units=off  parent_help=''  parent_units=''  use_min_max=off  parent_min=-inf  parent_max=inf  use_precision=off  parent_precision=''  parent_gain=1  parent_offset=0  parent_exp=1  use_mototune_group=on  parent_group='Sensors | Phoenix'
  motohawk_override_abs2 : MotoHawk_lib/Calibration & Probing Blocks/motohawk_override_abs  SystemSampleTime=-1  parent_name='Override_Absolute'  parent_val=0  show_more=on  name_source=Use Input Wire Name  parent_read_level=1  parent_override_level=1  view_as=Number  enum_struct={'Disabled', 'Enabled'}  use_help_units=off  parent_help=''  parent_units=''  use_min_max=off  parent_min=-inf  parent_max=inf  use_precision=off  parent_precision=''  parent_gain=1  parent_offset=0  parent_exp=1  use_mototune_group=on  parent_group='Sensors | Phoenix'
  motohawk_override_abs3 : MotoHawk_lib/Calibration & Probing Blocks/motohawk_override_abs  SystemSampleTime=-1  parent_name='DCVoltage_Phoenix'  parent_val=0  show_more=on  name_source=Use Parameter  parent_read_level=1  parent_override_level=1  view_as=Number  enum_struct={'Disabled', 'Enabled'}  use_help_units=off  parent_help=''  parent_units=''  use_min_max=off  parent_min=-inf  parent_max=inf  use_precision=off  parent_precision=''  parent_gain=1  parent_offset=0  parent_exp=1  use_mototune_group=on  parent_group='Sensors | Phoenix'
  motohawk_override_abs4 : MotoHawk_lib/Calibration & Probing Blocks/motohawk_override_abs  SystemSampleTime=-1  parent_name='SOC'  parent_val=0.5  show_more=on  name_source=Use Parameter  parent_read_level=1  parent_override_level=1  view_as=Number  enum_struct={'Disabled', 'Enabled'}  use_help_units=off  parent_help=''  parent_units=''  use_min_max=on  parent_min=0  parent_max=1  use_precision=off  parent_precision=''  parent_gain=1  parent_offset=0  parent_exp=1  use_mototune_group=on  parent_group='Sensors | BCM'
  motohawk_override_abs5 : MotoHawk_lib/Calibration & Probing Blocks/motohawk_override_abs  SystemSampleTime=-1  parent_name='bcm_ready'  parent_val=0  show_more=on  name_source=Use Parameter  parent_read_level=1  parent_override_level=1  view_as=Number  enum_struct={'Disabled', 'Enabled'}  use_help_units=off  parent_help=''  parent_units=''  use_min_max=off  parent_min=-inf  parent_max=inf  use_precision=off  parent_precision=''  parent_gain=1  parent_offset=0  parent_exp=1  use_mototune_group=on  parent_group='Sensors | BCM'
  motohawk_probe1 : MotoHawk_lib/Calibration & Probing Blocks/motohawk_probe  nam='DC_Voltage'  show_more=on  name_source=Use Parameter  read_level=1  view_as=Number  enum_struct={'Disabled', 'Enabled'}  vector_style=Wide Row  use_help_units=off  help=''  units=''  use_header_enum=off  row_header_enum={}  col_header_enum={}  use_precision=off  precision=''  gain=1  offset=0  exp=1  use_mototune_group=on  mototune_group='Sensors'
  motohawk_probe{2..4,9..10,46} (6 alike) : MotoHawk_lib/Calibration & Probing Blocks/motohawk_probe  nam='Probe'  show_more=on  name_source=Use Input Wire Name  read_level=1  view_as=Number  enum_struct={'Disabled', 'Enabled'}  vector_style=Wide Row  use_help_units=off  help=''  units=''  use_header_enum=off  row_header_enum={}  col_header_enum={}  use_precision=off  precision=''  gain=1  offset=0  exp=1  use_mototune_group=on  mototune_group='Sensors | Phoenix'
  motohawk_probe11 : MotoHawk_lib/Calibration & Probing Blocks/motohawk_probe  nam='BattMinTemp'  show_more=on  name_source=Use Parameter  read_level=1  view_as=Number  enum_struct={'Disabled', 'Enabled'}  vector_style=Wide Row  use_help_units=off  help=''  units=''  use_header_enum=off  row_header_enum={}  col_header_enum={}  use_precision=off  precision=''  gain=1  offset=0  exp=1  use_mototune_group=on  mototune_group='Sensors | Brusa'
  motohawk_probe12 : MotoHawk_lib/Calibration & Probing Blocks/motohawk_probe  nam='BattMaxTemp'  show_more=on  name_source=Use Parameter  read_level=1  view_as=Number  enum_struct={'Disabled', 'Enabled'}  vector_style=Wide Row  use_help_units=off  help=''  units=''  use_header_enum=off  row_header_enum={}  col_header_enum={}  use_precision=off  precision=''  gain=1  offset=0  exp=1  use_mototune_group=on  mototune_group='Sensors | Brusa'
  motohawk_probe{16..45} (30 alike) : MotoHawk_lib/Calibration & Probing Blocks/motohawk_probe  nam='Probe'  show_more=on  name_source=Use Input Wire Name  read_level=1  view_as=Number  enum_struct={'Disabled', 'Enabled'}  vector_style=Wide Row  use_help_units=off  help=''  units=''  use_header_enum=off  row_header_enum={}  col_header_enum={}  use_precision=off  precision=''  gain=1  offset=0  exp=1  use_mototune_group=on  mototune_group='Sensors | BCM'
  Sensors : Outport  OutDataType=sfix(16)  OutScaling=2^0
  wires:
  motohawk_ain/1 -> Linear Sensor Characterization/1(ADC)
  motohawk_ain1/1 -> Analog Switch/1
  Read CAN Message4/3 -> motohawk_override_abs1/1  "Motor_Speed"
  Read CAN Message4/4 -> motohawk_override_abs2/1  "Estimated_Motor_Torque"
  motohawk_override_abs2/1 -> motohawk_probe9/1, [motor_torque]  "Estimated_Motor_Torque"
  motohawk_override_abs1/1 -> motohawk_probe10/1, [motor_speed], Vehicle Speed/1(Motor_Speed)  "Motor_Speed"
  Read CAN Message2/1 -> Compare To Constant/1  "AgeCount"
  Analog Switch/1 -> [Brake_Sw]
  Linear Sensor Characterization/1(EngUnitsFilt) -> [Accel]
  Linear Sensor Characterization/2(EngUnitsRaw) -> Terminator2/1
  Bus Creator/1 -> Sensors/1
  [Accel] -> Bus Creator/1  "Accel"
  [Brake_Sw] -> Bus Creator/2  "BrakeSw"
  [Reverse_Sw] -> Bus Creator/3  "ReverseSw"
  motohawk_ain2/1 -> Analog Switch1/1
  Analog Switch1/1 -> [Reverse_Sw]
  motohawk_din/1 -> Analog Switch3/1
  Analog Switch3/1 -> [EStop_Sw], motohawk_fault_def3/1
  motohawk_ain5/1 -> Linear Sensor Characterization1/1
  Linear Sensor Characterization1/2 -> Terminator4/1
  motohawk_calibration3/1 -> Relational Operator3/2
  Linear Sensor Characterization1/1 -> [LVVoltage], Relational Operator3/1, Relational Operator4/1
  Relational Operator3/1 -> motohawk_fault_def5/1
  motohawk_calibration4/1 -> Relational Operator4/2
  Relational Operator4/1 -> motohawk_fault_def6/1
  Compare To Constant1/1 -> motohawk_fault_def1/1  "AgeCount"
  Compare To Constant/1 -> motohawk_fault_def/1  "AgeCount"
  Read CAN Message4/1 -> Compare To Constant1/1  "AgeCount"
  Read CAN Message4/2 -> Terminator/1
  Read CAN Message2/2 -> Terminator6/1
  Read CAN Message2/3 -> motohawk_override_abs3/1
  Read CAN Message3/1 -> Compare To Constant2/1  "AgeCount"
  Compare To Constant2/1 -> motohawk_fault_def9/1  "AgeCount"
  Read CAN Message3/2 -> Terminator7/1
  Read CAN Message3/3 -> motohawk_probe2/1  "Phoenix_Operating_State"
  Read CAN Message3/4 -> motohawk_probe3/1  "Phoenix_Operating_Mode"
  Read CAN Message3/5 -> motohawk_probe4/1  "Phoenix_Error"
  Read CAN Message1/2 -> motohawk_probe16/1  "bcm_alarm"
  Read CAN Message1/3 -> motohawk_probe17/1  "bcm_cpwr_cmd"
  Read CAN Message1/4 -> motohawk_probe18/1  "bcm_cpwr_mon"
  Read CAN Message1/5 -> motohawk_probe19/1  "bcm_epo"
  Read CAN Message1/6 -> motohawk_probe20/1, Relational Operator1/1  "bcm_gfd"
  Read CAN Message1/7 -> motohawk_probe21/1  "bcm_hvil_mon"
  Read CAN Message1/8 -> motohawk_probe22/1, [DC_Current]  "bcm_ibat"
  Read CAN Message1/9 -> motohawk_override_abs/1  "bcm_mainc_stat"
  Read CAN Message1/10 -> motohawk_override_abs5/1  "bcm_ready"
  Read CAN Message1/11 -> motohawk_probe25/1, Gain/1  "bcm_soc"
  Read CAN Message1/12 -> motohawk_probe26/1, [DC_Voltage], motohawk_probe1/1  "bcm_vbat"
  Read CAN Message1/13 -> motohawk_probe27/1  "bcm_chg_done"
  Read CAN Message1/14 -> motohawk_probe28/1  "bcm_chgc_stat"
  Read CAN Message1/15 -> motohawk_probe29/1  "bcm_cool_req"
  Read CAN Message5/2 -> motohawk_probe30/1  "bcm_cell_overvolt"
  Read CAN Message5/3 -> motohawk_probe31/1  "bcm_cell_undervolt"
  Read CAN Message5/4 -> motohawk_probe32/1  "bcm_chg_buf"
  Read CAN Message5/5 -> motohawk_probe33/1  "bcm_chg_max"
  Read CAN Message5/6 -> motohawk_probe34/1  "bcm_dis_buf"
  Read CAN Message5/7 -> motohawk_probe35/1  "bcm_dis_max"
  Read CAN Message5/8 -> motohawk_probe36/1  "bcm_t_coolant"
  Read CAN Message6/2 -> motohawk_probe37/1  "bcm_cell_tmax"
  Read CAN Message6/3 -> motohawk_probe38/1  "bcm_cell_tmin"
  Read CAN Message6/4 -> motohawk_probe39/1  "bcm_cell_vmax"
  Read CAN Message6/5 -> motohawk_probe40/1  "bcm_cell_vmin"
  Read CAN Message6/6 -> motohawk_probe41/1  "bcm_chga_ena"
  Read CAN Message6/7 -> motohawk_probe42/1  "bcm_chga_mon"
  Read CAN Message6/8 -> motohawk_probe43/1  "bcm_lvbat"
  Read CAN Message6/9 -> motohawk_probe44/1  "bcm_mod_ena"
  Read CAN Message6/10 -> motohawk_probe45/1  "bcm_veh_mon"
  Compare To Constant4/1 -> motohawk_fault_def10/1, Logical Operator1/1  "AgeCount"
  Read CAN Message1/1 -> Compare To Constant4/1  "AgeCount"
  Compare To Constant5/1 -> motohawk_fault_def11/1  "AgeCount"
  Read CAN Message5/1 -> Compare To Constant5/1  "AgeCount"
  Compare To Constant6/1 -> motohawk_fault_def12/1  "AgeCount"
  Read CAN Message6/1 -> Compare To Constant6/1  "AgeCount"
  Constant1/1 -> Relational Operator1/2
  motohawk_override_abs3/1 -> motohawk_probe46/1  "DC_Voltage_Phoenix"
  motohawk_override_abs4/1 -> [SOC]  "SOC"
  Gain/1 -> motohawk_override_abs4/1
  [DC_Current] -> Bus Creator/4  "DC_Current"
  [DC_Voltage] -> Bus Creator/5  "DC_Voltage"
  [motor_speed] -> Bus Creator/6  "MotorSpeed"
  [motor_torque] -> Bus Creator/7  "MotorTorque"
  [EStop_Sw] -> Bus Creator/8  "EStopSw"
  [LVVoltage] -> Bus Creator/9  "LVVoltage"
  [NLG5] -> Bus Creator/10  "NLG5"
  [SOC] -> Bus Creator/11  "SOC"
  Vehicle Speed/1(Vehicle_Speed) -> [VehicleSpeed]  "Vehicle_Speed"
  [VehicleSpeed] -> Bus Creator/12  "VehicleSpeed"
  Brusa Charger/1(Out1) -> [NLG5], Bus Selector1/1
  MinMax1/1 -> Relational Operator/1, motohawk_probe12/1
  motohawk_calibration/1 -> Relational Operator/2
  Relational Operator/1 -> motohawk_fault_def2/1
  MinMax/1 -> Relational Operator2/1, motohawk_probe11/1
  motohawk_calibration2/1 -> Relational Operator2/2
  Relational Operator2/1 -> motohawk_fault_def4/1
  Bus Selector1/1 -> Switch/2  "<TempSensExt1>"
  Bus Selector1/2 -> Switch/3  "<TempExtrn1>"
  Bus Selector1/3 -> Switch1/2  "<TempSensExt2>"
  Bus Selector1/4 -> Switch1/3  "<TempExtrn2>"
  Bus Selector1/5 -> Switch2/2  "<TempSensExt3>"
  Bus Selector1/6 -> Switch2/3  "<TempExtrn3>"
  Constant/1 -> Switch/1, Switch1/1, Switch2/1
  Switch/1 -> Mux/1
  Switch1/1 -> Mux/2
  Switch2/1 -> Mux/3
  Mux/1 -> MinMax/1, MinMax1/1
  [Contactor_Status] -> Bus Creator/14  "ContactorStatus"
  [Battery_Ready] -> Bus Creator/13  "BatteryReady"
  Relational Operator1/1 -> Logical Operator/2
  Logical Operator/1 -> motohawk_fault_def7/1
  Logical Operator1/1 -> Logical Operator/1
  motohawk_override_abs/1 -> motohawk_probe23/1, [Contactor_Status]  "bcm_mainc_stat"
  motohawk_override_abs5/1 -> [Battery_Ready], motohawk_probe24/1  "bcm_ready"

== system BuckyWagon_01/Main Power Relay/Background/Delay ==
  note: Delay the rising and falling of a boolean signal
  In : Inport  OutDataType=sfix(16)  OutScaling=2^0
  Constant1 : Constant  Value=0  OutDataType=sfix(16)  OutScaling=2^0  OutDataTypeStr=Inherit: Inherit via back propagation
  Constant2 : Constant  Value=uint16( on_delay_count )  OutDataType=sfix(16)  OutScaling=2^0
  Constant3 : Constant  Value=0  OutDataType=sfix(16)  OutScaling=2^0  OutDataTypeStr=Inherit: Inherit via back propagation
  Constant4 : Constant  Value=uint16( off_delay_count )  OutDataType=sfix(16)  OutScaling=2^0
  Data Type Conversion : DataTypeConversion  RndMeth=Zero
  Data Type Conversion1 : DataTypeConversion  RndMeth=Zero
  Logical Operator : Logic  Operator=NOT  OutDataTypeMode=boolean  OutDataTypeStr=boolean
  Logical Operator1 : Logic  OutDataTypeMode=boolean  OutDataTypeStr=boolean
  Logical Operator2 : Logic  OutDataTypeMode=boolean  OutDataTypeStr=boolean
  MotoHawk S-R Flip-Flop : Subsystem  mask(MotoHawk S-R Flip-Flop){ic_bool=false}
      mask prompts: ic_bool "Initial condition Q (boolean)"
      mask help:
      | When input S (set) is TRUE, output Q is TRUE (and latched until reset).
      | When input R (reset) is TRUE, output Q is FALSE (and latched until set).
      | If both inputs S and R are TRUE, output Q is FALSE (reset wins).
      mask Display:
      | patch([0 0 1 1], [0 0.075 0.075 0], [230/255 0/255 0/255]);
      | patch([0 0 1 1], [0.025 0.05 0.05 0.025], [150/255 0/255 0/255]);
      | patch([0 0 1 1], [0 0.025 0.025 0], [0/255 0/255 0/255])
  Relational Operator1 : RelationalOperator  LogicOutDataTypeMode=boolean  OutDataTypeStr=boolean  ZeroCross=off  InputSameDT=on
  Relational Operator2 : RelationalOperator  LogicOutDataTypeMode=boolean  OutDataTypeStr=boolean  ZeroCross=off  InputSameDT=on
  Sum : Sum  Inputs=++|  OutDataType=sfix(16)  OutScaling=2^0  RndMeth=Zero  SaturateOnIntegerOverflow=on  InputSameDT=on
  Sum1 : Sum  Inputs=++|  OutDataType=sfix(16)  OutScaling=2^0  RndMeth=Zero  SaturateOnIntegerOverflow=on  InputSameDT=on
  Switch : Switch  Criteria=u2 ~= 0  Threshold=1  RndMeth=Zero  ZeroCross=off  InputSameDT=on
  Switch1 : Switch  Criteria=u2 ~= 0  Threshold=1  RndMeth=Zero  ZeroCross=off  InputSameDT=on
  Terminator : Terminator
  Unit Delay : UnitDelay  SampleTime=-1
  Unit Delay1 : UnitDelay  SampleTime=-1
  Out : Outport
  wires:
  Logical Operator1/1 -> MotoHawk S-R Flip-Flop/2(R)
  Logical Operator2/1 -> MotoHawk S-R Flip-Flop/1(S)
  Relational Operator1/1 -> Logical Operator2/2
  Relational Operator2/1 -> Logical Operator1/2
  MotoHawk S-R Flip-Flop/2(!Q) -> Terminator/1
  MotoHawk S-R Flip-Flop/1(Q) -> Out/1
  Constant4/1 -> Relational Operator2/2
  Logical Operator/1 -> Logical Operator1/1, Switch1/2, Data Type Conversion1/1
  Data Type Conversion1/1 -> Sum1/2  "0 to 1"
  Sum1/1 -> Switch1/1  "0 to 65535 (saturate hi)"
  Constant3/1 -> Switch1/3
  Switch1/1 -> Relational Operator2/1, Unit Delay1/1  "0 to 65535"
  In/1 -> Logical Operator/1, Logical Operator2/1, Switch/2, Data Type Conversion/1
  Data Type Conversion/1 -> Sum/2  "0 to 1"
  Sum/1 -> Switch/1  "0 to 65535 (saturate hi)"
  Constant1/1 -> Switch/3
  Switch/1 -> Unit Delay/1, Relational Operator1/1  "0 to 65535"
  Constant2/1 -> Relational Operator1/2
  Unit Delay1/1 -> Sum1/1  "0 to 65535"
  Unit Delay/1 -> Sum/1  "0 to 65535"

== system BuckyWagon_01/Main Power Relay/Background/Post Shutdown two ticks before MPRD off ==
  Trigger : TriggerPort  TriggerType=falling
  Function-Call Generator : simulink/Ports & Subsystems/Function-Call Generator  sample_time=-1  numberOfIterations=1
  Post Shutdown two ticks before MPRD off : MotoHawk_lib/Trigger Blocks/motohawk_event_call  SystemSampleTime=-1  mode=Post Event  trigger=SHUTDOWN_EVENT  target=ECU565_128
  motohawk_code_coverage : MotoHawk_lib/Extra Development Blocks/motohawk_code_coverage
  wires:
  Function-Call Generator/1 -> Post Shutdown two ticks before MPRD off/Trigger

== system BuckyWagon_01/Main Power Relay/Background/Processor Reboot ==
  Enable : EnablePort
  Trigger : TriggerPort  TriggerType=falling
  Force Module Reset : MotoHawk_lib/Extra Development Blocks/Force Module Reset
  motohawk_code_coverage : MotoHawk_lib/Extra Development Blocks/motohawk_code_coverage

== system BuckyWagon_01/Main Power Relay/Background/Save NV Vars one tick before MPRD off ==
  Trigger : TriggerPort  TriggerType=falling
  Function-Call Generator : simulink/Ports & Subsystems/Function-Call Generator  sample_time=-1  numberOfIterations=1
  Save NV Vars one tick before MPRD off : MotoHawk_lib/Data Storage Blocks/motohawk_store_nvmem  SystemSampleTime=-1
  motohawk_code_coverage : MotoHawk_lib/Extra Development Blocks/motohawk_code_coverage
  wires:
  Function-Call Generator/1 -> Save NV Vars one tick before MPRD off/Trigger
